simulink model "control_model22"  (R2018a)
settings: Solver=ode3  StartTime=0.0  StopTime=50  FixedStep=Te
InitFcn:
  | Tp=60
values from neighbouring files (symbols this model uses):
  den = [a2 a1 a0]    [transfer_function.m]
  f = 0.0001    [IM_model.m]    (also in transfer_function.m)
  J = 0.011    [IM_model.m]    (also in transfer_function.m)
  Lr = 0.0302409    [IM_model.m]    (also in transfer_function.m)
  Ls = 0.0302409    [IM_model.m]    (also in transfer_function.m)
  num = [K]    [transfer_function.m]
  p = 1    [IM_model.m]    (also in transfer_function.m)
  Rr = 10.3654    [IM_model.m]    (also in transfer_function.m)
  Rs = 11    [IM_model.m]    (also in transfer_function.m)
  Te = 10^-4    (= 0.0001)    [IM_model.m]    (also in data_aquisition11.m = 0.001)
libraries: neural x21, powerlib x15, peGeneralControl x9, pePwmGenerator x3, simulink x2, powerlib_meascontrol x2
(part 2 of 2)

== matlab function control_model22/MATLAB Function ==
  data: ref output; t input
function ref = reference_signal(t)
    max_val = 2950;
    min_val = 1200;
    dur = 12;  
     N = 10;    
 
    full_range = max_val - min_val;
    step_size = full_range / N;
    slew_rate = 0.1 * full_range;  % 10% of full range per second
    
    t_ramp = step_size / slew_rate;   % ramp duration per step
    t_hold = dur - t_ramp;             % hold duration per step
    
    total_steps = 2 * N;
    
    step_index = floor(t / dur);
    t_in_step = mod(t, dur);
    
    if step_index < N
        % Ramp up phase
        start_val = min_val + step_index * step_size;
        end_val = start_val + step_size;
    elseif step_index < total_steps
        % Ramp down phase
        descending_index = step_index - N;
        start_val = max_val - descending_index * step_size;
        end_val = start_val - step_size;
    else
        % After all steps, hold at min_val
        ref = min_val;
        return;
    end
    
    if t_in_step < t_ramp
        % Ramp phase: linear interpolation
        ref = start_val + (end_val - start_val) * (t_in_step / t_ramp);
    else
        % Hold phase: constant value
        ref = end_val;
    end
end

== matlab function control_model22/Driving circuit/MATLAB Function ==
  data: wt input; va output; vb output; vc output
function [va, vb, vc] = ThreePhaseSine(wt)

    va = sin(wt);
    vb = sin(wt - 2*pi/3);
    vc = sin(wt - 4*pi/3);
end

== matlab function control_model22/MATLAB Function1 ==
  data: ref output; t input
function ref = reference_signal(t)
    max_val = 0.5;
    min_val = 0;
    dur = 6;    % total duration per step (ramp + hold)
    N = 20;     % number of steps for each ramp (up and down)
    
    full_range = max_val - min_val;
    step_size = full_range / N;
    slew_rate = 0.1 * full_range;  % 10% of full range per second
    
    t_ramp = step_size / slew_rate;   % ramp duration per step
    t_hold = dur - t_ramp;             % hold duration per step
    
    total_steps = 2 * N;
    
    step_index = floor(t / dur);
    t_in_step = mod(t, dur);
    
    if step_index < N
        % Ramp up phase
        start_val = min_val + step_index * step_size;
        end_val = start_val + step_size;
    elseif step_index < total_steps
        % Ramp down phase
        descending_index = step_index - N;
        start_val = max_val - descending_index * step_size;
        end_val = start_val - step_size;
    else
        % After all steps, hold at min_val
        ref = min_val;
        return;
    end
    
    if t_in_step < t_ramp
        % Ramp phase: linear interpolation between start_val and end_val
        ref = start_val + (end_val - start_val) * (t_in_step / t_ramp);
    else
        % Hold phase: constant at end_val
        ref = end_val;
    end
end
